simulink model "LQRSim_Goal_1"  (R2020a)
settings: Solver=VariableStepAuto  StartTime=0.0  StopTime=2  RelTol=1e-3
values from neighbouring files (symbols this model uses):
  Ix = 4.856*10^-3    (= 0.004856)    [LQR.m]    (also in LQR_Goal_1.m; Naman_LQR_Working.m; PlantModel.m)
  Iy = 4.856*10^-3    (= 0.004856)    [LQR.m]    (also in LQR_Goal_1.m; Naman_LQR_Working.m; PlantModel.m)
  Iz = 8.801*10^-3    (= 0.008801)    [LQR.m]    (also in LQR_Goal_1.m; Naman_LQR_Working.m; PlantModel.m)
  K = zeros(length(R), length(Q), nSteps)    [LQR.m]    (also in LQR_Goal_1.m; Naman_LQR_Working.m)
  m = 0.468    [LQR.m]    (also in LQR_Goal_1.m; Naman_LQR_Working.m; PlantModel.m)
  T_s = 0.05    [LQR.m]    (also in LQR_Goal_1.m = 0.01; Naman_LQR_Working.m = 0.01)
  x_0_up = [0, 0, -1,            0, 0, 0,            0, 0, 0,            0, 0, 0]'    [LQR.m]    (also in LQR_Goal_1.m = [0, 0, -1,         0, 0, 0,         0, 0, 0,         0, 0, 0; Naman_LQR_Working.m = [0, 0, -1,         0, 0, 0,         0, 0, 0,         0, 0, 0)
libraries: simulink x1
settings Model: Creator=Lakshu  LastModifiedBy=Sravan

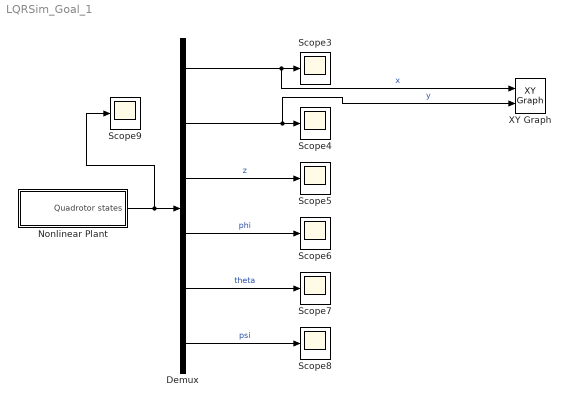
== system LQRSim_Goal_1 ==
  Demux : Demux  Outputs=6
  Nonlinear Plant : Subsystem
  Scope{3..9} (7 alike) : Scope
  XY Graph : simulink/Sinks/XY Graph  xmin=-7  xmax=7  ymin=-7  ymax=7  st=-1
  wires:
  Nonlinear Plant/1(Quadrotor states) -> Scope9/1, Demux/1
  Demux/1 -> XY Graph/1, Scope3/1  "x"
  Demux/2 -> XY Graph/2, Scope4/1  "y"
  Demux/3 -> Scope5/1  "z"
  Demux/4 -> Scope6/1  "phi"
  Demux/5 -> Scope7/1  "theta"
  Demux/6 -> Scope8/1  "psi"

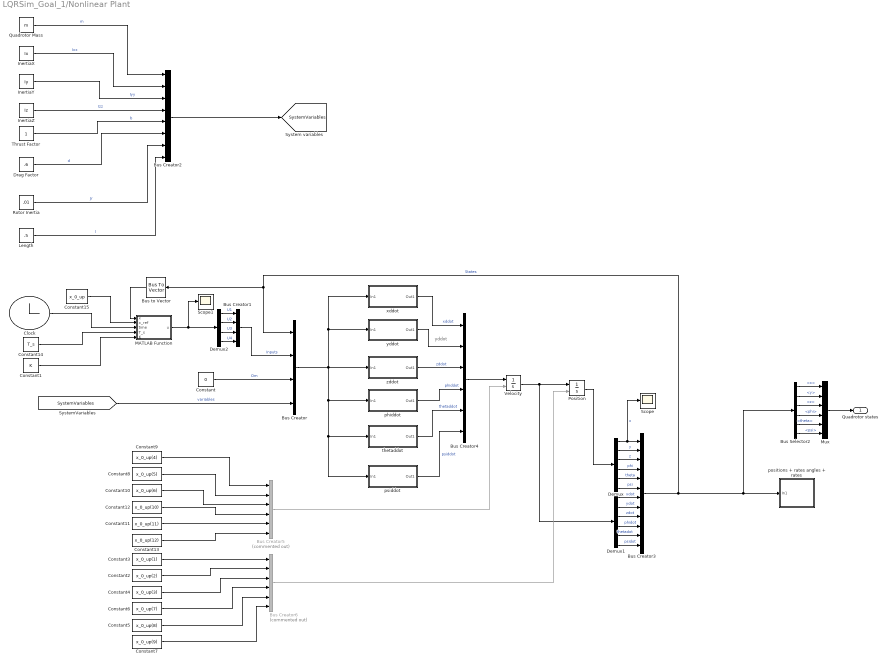
== system LQRSim_Goal_1/Nonlinear Plant ==
  note: yddot
  Bus Creator : BusCreator  Inputs=4
  Bus Creator1 : BusCreator  Inputs=4
  Bus Creator2 : BusCreator  Inputs=8
  Bus Creator3 : BusCreator  Inputs=12
  Bus Creator4 : BusCreator  Inputs=6
  Bus Creator5 : BusCreator  Commented=on  Inputs=6
  Bus Creator6 : BusCreator  Commented=on  Inputs=6
  Bus Selector2 : BusSelector  OutputSignals=x,y,z,phi,theta,psi
  Bus to Vector : BusToVector
  Clock : Clock
  Constant : Constant  Value=0
  Constant1 : Constant  Value=K
  Constant10 : Constant  Value=x_0_up(6)
  Constant11 : Constant  Value=x_0_up(11)
  Constant12 : Constant  Value=x_0_up(10)
  Constant13 : Constant  Value=x_0_up(12)
  Constant14 : Constant  Value=T_s
  Constant15 : Constant  Value=x_0_up
  Constant2 : Constant  Value=x_0_up(2)
  Constant3 : Constant  Value=x_0_up(1)
  Constant4 : Constant  Value=x_0_up(3)
  Constant5 : Constant  Value=x_0_up(8)
  Constant6 : Constant  Value=x_0_up(7)
  Constant7 : Constant  Value=x_0_up(9)
  Constant8 : Constant  Value=x_0_up(5)
  Constant9 : Constant  Value=x_0_up(4)
  Demux : Demux  Outputs=6
  Demux1 : Demux  Outputs=6
  Demux2 : Demux
  Drag Factor : Constant  Value=.6
  InertiaX : Constant  Value=Ix
  InertiaY : Constant  Value=Iy
  InertiaZ : Constant  Value=Iz
  Length : Constant  Value=.5
  MATLAB Function : MATLAB Function  TreatAsAtomicUnit=on
  Mux : Mux  Inputs=6
  Position : Integrator  InitialConditionSource=external
  Quadrotor Mass : Constant  Value=m
  Rotor Inertia : Constant  Value=.01
  Scope : Scope
  Scope1 : Scope
  Thrust Factor : Constant
  Velocity : Integrator  InitialConditionSource=external
  phiddot : Subsystem
  positions + rates angles + rates : Subsystem
      mask Display: disp('system states')
  psiddot : Subsystem
  thetaddot : Subsystem
  xddot : Subsystem
  yddot : Subsystem
  zddot : Subsystem
  Quadrotor states : Outport
  tag scope: SystemVariables=global
  wires:
  [SystemVariables] -> Bus Creator/4  "variables"
  Bus Creator/1 -> xddot/1(In1), yddot/1(In1), zddot/1(In1), phiddot/1(In1), thetaddot/1(In1), psiddot/1(In1)
  xddot/1(Out1) -> Bus Creator4/1  "xddot"
  yddot/1(Out1) -> Bus Creator4/2
  zddot/1(Out1) -> Bus Creator4/3  "zddot"
  phiddot/1(Out1) -> Bus Creator4/4  "phiddot"
  thetaddot/1(Out1) -> Bus Creator4/5  "thetaddot"
  psiddot/1(Out1) -> Bus Creator4/6  "psiddot"
  Position/1 -> Demux/1
  Bus Creator4/1 -> Velocity/1
  Velocity/1 -> Position/1, Demux1/1
  Constant9/1 -> Bus Creator5/1
  Constant8/1 -> Bus Creator5/2
  Constant10/1 -> Bus Creator5/3
  Constant12/1 -> Bus Creator5/4
  Constant11/1 -> Bus Creator5/5
  Constant13/1 -> Bus Creator5/6
  Bus Creator5/1 -> Velocity/2
  Constant3/1 -> Bus Creator6/1
  Constant2/1 -> Bus Creator6/2
  Constant4/1 -> Bus Creator6/3
  Constant6/1 -> Bus Creator6/4
  Constant5/1 -> Bus Creator6/5
  Constant7/1 -> Bus Creator6/6
  Bus Creator6/1 -> Position/2
  Demux/1 -> Scope/1, Bus Creator3/1  "x"
  Demux/2 -> Bus Creator3/2  "y"
  Demux/3 -> Bus Creator3/3  "z"
  Demux/4 -> Bus Creator3/4  "phi"
  Demux/5 -> Bus Creator3/5  "theta"
  Demux/6 -> Bus Creator3/6  "psi"
  Demux1/1 -> Bus Creator3/7  "xdot"
  Demux1/2 -> Bus Creator3/8  "ydot"
  Demux1/3 -> Bus Creator3/9  "zdot"
  Demux1/4 -> Bus Creator3/10  "phidot"
  Demux1/5 -> Bus Creator3/11  "thetadot"
  Demux1/6 -> Bus Creator3/12  "psidot"
  Bus Creator3/1 -> Bus Selector2/1, positions + rates angles + rates/1(In1), Bus Creator/1, Bus to Vector/1  "States"
  Rotor Inertia/1 -> Bus Creator2/7  "Jr"
  Length/1 -> Bus Creator2/8  "l"
  InertiaX/1 -> Bus Creator2/2  "Ixx"
  Drag Factor/1 -> Bus Creator2/6  "d"
  Quadrotor Mass/1 -> Bus Creator2/1  "m"
  Bus Creator2/1 -> [SystemVariables]
  InertiaZ/1 -> Bus Creator2/4  "Izz"
  InertiaY/1 -> Bus Creator2/3  "Iyy"
  Thrust Factor/1 -> Bus Creator2/5  "b"
  Constant/1 -> Bus Creator/3  "Om"
  Bus Selector2/1 -> Mux/1  "<x>"
  Bus Selector2/2 -> Mux/2  "<y>"
  Bus Selector2/3 -> Mux/3  "<z>"
  Bus Selector2/4 -> Mux/4  "<phi>"
  Bus Selector2/5 -> Mux/5  "<theta>"
  Bus Selector2/6 -> Mux/6  "<psi>"
  Mux/1 -> Quadrotor states/1
  Clock/1 -> MATLAB Function/3(time)
  Constant1/1 -> MATLAB Function/5(K)
  Bus Creator1/1 -> Bus Creator/2  "Inputs"
  Demux2/1 -> Bus Creator1/1  "U1"
  Demux2/2 -> Bus Creator1/2  "U2"
  Demux2/3 -> Bus Creator1/3  "U3"
  Demux2/4 -> Bus Creator1/4  "U4"
  MATLAB Function/1(u) -> Scope1/1, Demux2/1
  Bus to Vector/1 -> MATLAB Function/1(x)
  Constant14/1 -> MATLAB Function/4(T_s)
  Constant15/1 -> MATLAB Function/2(x_ref)

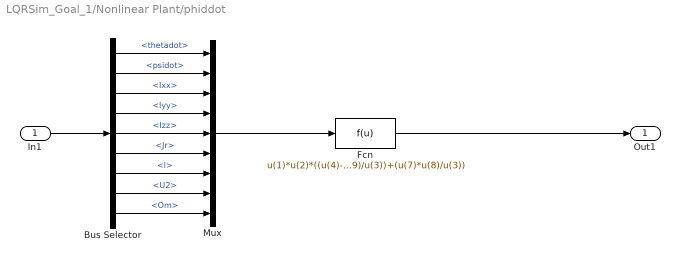
== system LQRSim_Goal_1/Nonlinear Plant/phiddot ==
  In1 : Inport
  Bus Selector : BusSelector  OutputSignals=States.thetadot,States.psidot,variables.Ixx,variables.Iyy,variables.Izz,variables.Jr,variables.l,Inputs.U2,Om
  Fcn : Fcn  Expr=u(1)*u(2)*((u(4)-u(5))/u(3))-(u(6)*u(1)*u(9)/u(3))+(u(7)*u(8)/u(3))
  Mux : Mux  Inputs=9
  Out1 : Outport
  wires:
  Bus Selector/7 -> Mux/7  "<l>"
  Mux/1 -> Fcn/1
  Bus Selector/3 -> Mux/3  "<Ixx>"
  Bus Selector/8 -> Mux/8  "<U2>"
  Bus Selector/5 -> Mux/5  "<Izz>"
  Bus Selector/4 -> Mux/4  "<Iyy>"
  Bus Selector/2 -> Mux/2  "<psidot>"
  Bus Selector/1 -> Mux/1  "<thetadot>"
  In1/1 -> Bus Selector/1
  Bus Selector/9 -> Mux/9  "<Om>"
  Fcn/1 -> Out1/1
  Bus Selector/6 -> Mux/6  "<Jr>"

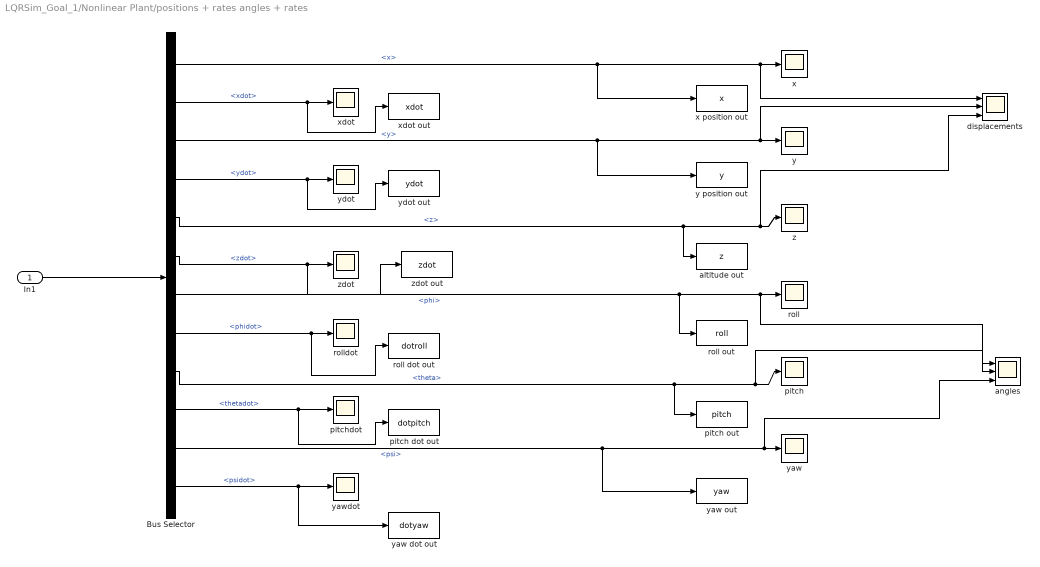
== system LQRSim_Goal_1/Nonlinear Plant/positions + rates angles + rates ==
  In1 : Inport
  Bus Selector : BusSelector  OutputSignals=x,xdot,y,ydot,z,zdot,phi,phidot,theta,thetadot,psi,psidot
  altitude out : ToWorkspace  VariableName=z  SampleTime=-1
  angles : Scope  NumInputPorts=3
  displacements : Scope  NumInputPorts=3
  pitch : Scope
  pitch dot out : ToWorkspace  VariableName=dotpitch  SampleTime=-1
  pitch out : ToWorkspace  VariableName=pitch  SampleTime=-1
  pitchdot : Scope
  roll : Scope
  roll dot out : ToWorkspace  VariableName=dotroll  SampleTime=-1
  roll out : ToWorkspace  VariableName=roll  SampleTime=-1
  rolldot : Scope
  x : Scope
  x position out : ToWorkspace  VariableName=x  SampleTime=-1
  xdot : Scope
  xdot out : ToWorkspace  VariableName=xdot  SampleTime=-1
  y : Scope
  y position out : ToWorkspace  VariableName=y  SampleTime=-1
  yaw : Scope
  yaw dot out : ToWorkspace  VariableName=dotyaw  SampleTime=-1
  yaw out : ToWorkspace  VariableName=yaw  SampleTime=-1
  yawdot : Scope
  ydot : Scope
  ydot out : ToWorkspace  VariableName=ydot  SampleTime=-1
  z : Scope
  zdot : Scope
  zdot out : ToWorkspace  VariableName=zdot  SampleTime=-1
  wires:
  Bus Selector/2 -> xdot/1, xdot out/1  "<xdot>"
  Bus Selector/4 -> ydot/1, ydot out/1  "<ydot>"
  Bus Selector/1 -> x position out/1, x/1, displacements/1  "<x>"
  Bus Selector/3 -> y position out/1, y/1, displacements/2  "<y>"
  Bus Selector/12 -> yawdot/1, yaw dot out/1  "<psidot>"
  Bus Selector/11 -> yaw out/1, yaw/1, angles/3  "<psi>"
  In1/1 -> Bus Selector/1
  Bus Selector/10 -> pitchdot/1, pitch dot out/1  "<thetadot>"
  Bus Selector/5 -> altitude out/1, z/1, displacements/3  "<z>"
  Bus Selector/6 -> zdot/1, zdot out/1  "<zdot>"
  Bus Selector/7 -> roll out/1, roll/1, angles/1  "<phi>"
  Bus Selector/8 -> rolldot/1, roll dot out/1  "<phidot>"
  Bus Selector/9 -> pitch out/1, pitch/1, angles/2  "<theta>"

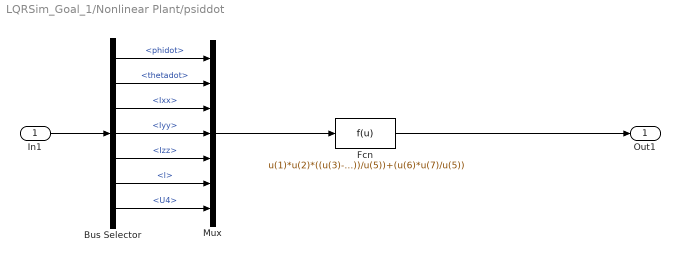
== system LQRSim_Goal_1/Nonlinear Plant/psiddot ==
  In1 : Inport
  Bus Selector : BusSelector  OutputSignals=States.phidot,States.thetadot,variables.Ixx,variables.Iyy,variables.Izz,variables.l,Inputs.U4
  Fcn : Fcn  Expr=u(1)*u(2)*((u(3)-u(4))/u(5))+(u(6)*u(7)/u(5))
  Mux : Mux  Inputs=7
  Out1 : Outport
  wires:
  Fcn/1 -> Out1/1
  Mux/1 -> Fcn/1
  In1/1 -> Bus Selector/1
  Bus Selector/1 -> Mux/1  "<phidot>"
  Bus Selector/2 -> Mux/2  "<thetadot>"
  Bus Selector/3 -> Mux/3  "<Ixx>"
  Bus Selector/4 -> Mux/4  "<Iyy>"
  Bus Selector/5 -> Mux/5  "<Izz>"
  Bus Selector/6 -> Mux/6  "<l>"
  Bus Selector/7 -> Mux/7  "<U4>"

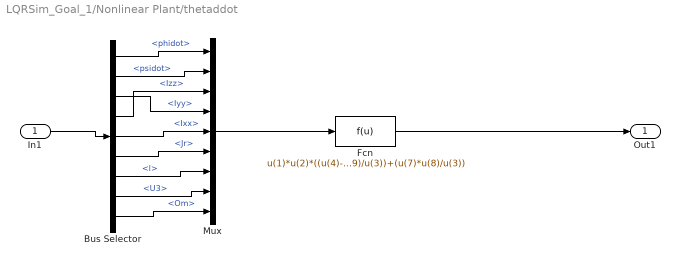
== system LQRSim_Goal_1/Nonlinear Plant/thetaddot ==
  In1 : Inport
  Bus Selector : BusSelector  OutputSignals=States.phidot,States.psidot,variables.Iyy,variables.Izz,variables.Ixx,variables.Jr,variables.l,Inputs.U3,Om
  Fcn : Fcn  Expr=u(1)*u(2)*((u(4)-u(5))/u(3))+(u(6)*u(1)*u(9)/u(3))+(u(7)*u(8)/u(3))
  Mux : Mux  Inputs=9
  Out1 : Outport
  wires:
  Bus Selector/1 -> Mux/1  "<phidot>"
  Bus Selector/2 -> Mux/2  "<psidot>"
  Bus Selector/7 -> Mux/7  "<l>"
  Bus Selector/6 -> Mux/6  "<Jr>"
  Bus Selector/3 -> Mux/4  "<Iyy>"
  In1/1 -> Bus Selector/1
  Mux/1 -> Fcn/1
  Fcn/1 -> Out1/1
  Bus Selector/4 -> Mux/3  "<Izz>"
  Bus Selector/5 -> Mux/5  "<Ixx>"
  Bus Selector/8 -> Mux/8  "<U3>"
  Bus Selector/9 -> Mux/9  "<Om>"

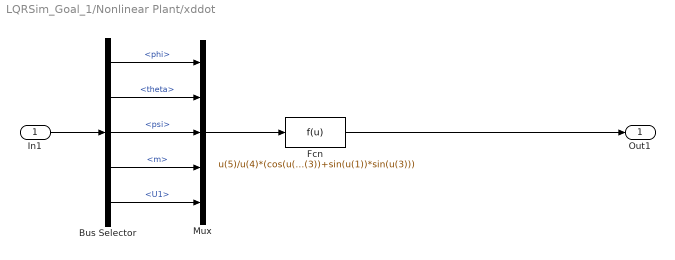
== system LQRSim_Goal_1/Nonlinear Plant/xddot ==
  In1 : Inport
  Bus Selector : BusSelector  OutputSignals=States.phi,States.theta,States.psi,variables.m,Inputs.U1
  Fcn : Fcn  Expr=u(5)/u(4)*(cos(u(1))*sin(u(2))*cos(u(3))+sin(u(1))*sin(u(3)))
  Mux : Mux  Inputs=5
  Out1 : Outport
  wires:
  In1/1 -> Bus Selector/1
  Bus Selector/1 -> Mux/1  "<phi>"
  Bus Selector/2 -> Mux/2  "<theta>"
  Bus Selector/3 -> Mux/3  "<psi>"
  Bus Selector/4 -> Mux/4  "<m>"
  Bus Selector/5 -> Mux/5  "<U1>"
  Mux/1 -> Fcn/1
  Fcn/1 -> Out1/1

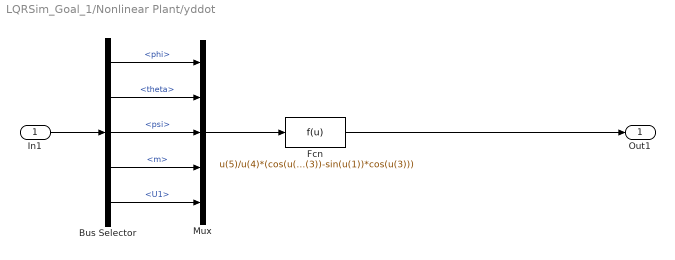
== system LQRSim_Goal_1/Nonlinear Plant/yddot ==
  In1 : Inport
  Bus Selector : BusSelector  OutputSignals=States.phi,States.theta,States.psi,variables.m,Inputs.U1
  Fcn : Fcn  Expr=u(5)/u(4)*(cos(u(1))*sin(u(2))*sin(u(3))-sin(u(1))*cos(u(3)))
  Mux : Mux  Inputs=5
  Out1 : Outport
  wires:
  Fcn/1 -> Out1/1
  Mux/1 -> Fcn/1
  Bus Selector/5 -> Mux/5  "<U1>"
  Bus Selector/4 -> Mux/4  "<m>"
  Bus Selector/3 -> Mux/3  "<psi>"
  Bus Selector/2 -> Mux/2  "<theta>"
  Bus Selector/1 -> Mux/1  "<phi>"
  In1/1 -> Bus Selector/1

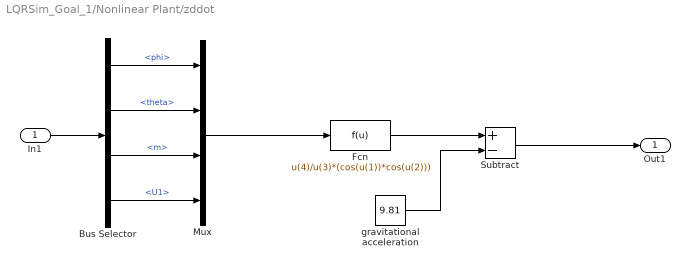
== system LQRSim_Goal_1/Nonlinear Plant/zddot ==
  In1 : Inport
  Bus Selector : BusSelector  OutputSignals=States.phi,States.theta,variables.m,Inputs.U1
  Fcn : Fcn  Expr=u(4)/u(3)*(cos(u(1))*cos(u(2)))
  Mux : Mux
  Subtract : Sum  Inputs=+-
  gravitational acceleration : Constant  Value=9.81
  Out1 : Outport
  wires:
  In1/1 -> Bus Selector/1
  Bus Selector/1 -> Mux/1  "<phi>"
  Bus Selector/2 -> Mux/2  "<theta>"
  Mux/1 -> Fcn/1
  Bus Selector/3 -> Mux/3  "<m>"
  Bus Selector/4 -> Mux/4  "<U1>"
  Fcn/1 -> Subtract/1
  gravitational acceleration/1 -> Subtract/2
  Subtract/1 -> Out1/1

== matlab function LQRSim_Goal_1/Nonlinear Plant/MATLAB Function ==
  data: x input; x_ref input; time input; T_s input; u output; K input
function u = fcn(x, x_ref, time, T_s, K)
    i = floor(time/T_s) + 1;
    state = x + x_ref;
    u = K(:,:,i) * state;
end
